simulink model "DrivetrainConVeh"  (R2024a)
settings: Solver=ode23tb  StartTime=0.0  StopTime=50  RelTol=1e-3  EnableMultiTasking=on
model workspace (MAT data in the model file):
  N : Simulink.Parameter (value not decoded)
  NF : Simulink.Parameter (value not decoded)
  NR : Simulink.Parameter (value not decoded)
  Ndiff : Simulink.Parameter (value not decoded)
  RWheel : Simulink.Parameter (value not decoded)
  b_axle : Simulink.Parameter (value not decoded)
  b_driveshaft : Simulink.Parameter (value not decoded)
  dt_DCT : Simulink.Parameter (value not decoded)
  k_axle : Simulink.Parameter (value not decoded)
  k_driveshaft : Simulink.Parameter (value not decoded)
  k_hyd : Simulink.Parameter (value not decoded)
  tau_hyd : Simulink.Parameter (value not decoded)
  wc_shaft : Simulink.Parameter (value not decoded)
symbols that are objects in the model workspace (value not decoded): b_axle, b_driveshaft, k_axle, k_driveshaft, k_hyd, N, tau_hyd
libraries: autolibsharedcoupling x12, autolibpowerinfoutils x6, autolibshareddiff x5, autolibutils x3, autolibshared x3, autolibcoupling x2, simulink x2, autolibsharedtransfixedgear x2, autolibtransdct x1, autolibshareddrivetraincommon x1, autolibtranscontrols x1
(part 3 of 4)

== system DrivetrainConVeh/DCT/DCT Block ==
  GearReq : Inport
  Tin : Inport  Port=2
  Driveshaft Compliance : autolibsharedcoupling/Torsional Compliance  port_config=Two-way connection  extInfo=off  k=k_driveshaft  b=b_driveshaft  theta_o=0  domega_o=0  omega_c=wc_shaft  blkID=0  aMode=1
  Dual Clutch Transmission : autolibtransdct/Dual Clutch Transmission  VariantControl=0  cntrlType=Ideal integrated controller  TransEffModelPopup=Gear only  Jin=0.2  bin=.001  omegain_o=0  G=[-1, 0, 1, 2, 3, 4, 5, 6, 7, 8]  Trq_bpts=[25 50 75 100 150 200 250]  omega_bpts=[52.4 78.5 105 131 157 183 209 262 314 419 524]  Temp_bpts=[313 358]  N=N  Jout=[0.28 0.28 0.28 0.24 0.2 0.18 0.11 0.11 0.11 0.11]  bout=[.001 .001 .001 .0025 .002 .001 .001 .001 .001 .001]  eta=[0.930, 0.930, 0.930, 0.940,0.947, 0.948,0.946, 0.943,0.940, 0.935 ]  eta_tbl=reshape([0.57 0.77 0.83 0.86 0.89 0.89 0.89 0.55 0.76 0.83 0.86 0.89 0.89 0.89 0.59 0.78 0.85 0.88 0.9 0.89 0.89 0.61 0.79 0.85 0.88 0.91 0.89 0.89 0.62 0.8 0.86 0.89 0.91 0.89 0.89 0.62 0.8 0.85 0.89 0.91 0.89 0.89 0.63 0.8 0.86 0.89 0.92 0.89 0.89 0.63 0.8 0.86 0.89 0.92 0.89 0.89 0.62 0.81 0.86 0.89 0.92 0.89 0.89 0.6 0.79 0.85 0.88 0.92 0.89 0.89 0.55 0.77 0.84 0.87 0.91 0.89 0.89 0.57 0.77 0.83 0.86 0.89 0.89 0.89 0.55 0.76 0.83 0.86 0.89 0.89 0.89 0.59 0.78 0.85 0.88 0.9 0.89 0.89 0.61 0.79 0.85 0.88 0.91 0.89 0.89 0.62 0.8 0.86 0.89 0.91 0.89 0.89 0.62 0.8 0.85 0.89 0.91 0.89 0.89 0.63 0.8 0.86 0.89 0.92 0.89 0.89 0.63 0.8 0.86 0.89 0.92 0.89 0.89 0.62 0.81 0.86 0.89 0.92 0.89 0.89 0.6 0.79 0.85 0.88 0.92 0.89 0.89 0.55 0.77 0.84 0.87 0.91 0.89 0.89 0.57 0.77 0.83 0.86 0.89 0.89 0.89 0.55 0.76 0.83 0.86 0.89 0.89 0.89 0.59 0.78 0.85 0.88 0.9 0.89 0.89 0.61 0.79 0.85 0.88 0.91 0.89 0.89 0.62 0.8 0.86 0.89 0.91 0.89 0.89 0.62 0.8 0.85 0.89 0.91 0.89 0.89 0.63 0.8 0.86 0.89 0.92 0.89 0.89 0.63 0.8 0.86 0.89 0.92 0.89 0.89 0.62 0.81 0.86 0.89 0.92 0.89 0.89 0.6 0.79 0.85 0.88 0.92 0.89 0.89 0.55 0.77 0.84 0.87 0.91 0.89 0.89 0.76 0.87 0.9 0.91 0.93 0.92 0.92 0.69 0.83 0.88 0.9 0.91 0.92 0.92 0.64 0.81 0.87 0.89 0.91 0.92 0.92 0.63 0.81 0.86 0.89 0.91 0.92 0.92 0.63 0.81 0.86 0.89 0.92 0.92 0.92 0.62 0.8 0.86 0.89 0.92 0.93 0.92 0.62 0.8 0.86 0.89 0.92 0.93 0.92 0.61 0.8 0.86 0.89 0.92 0.93 0.92 0.61 0.8 0.86 0.89 0.92 0.93 0.92 0.57 0.78 0.84 0.88 0.91 0.93 0.92 0.52 0.76 0.83 0.87 0.91 0.93 0.92 0.71 0.84 0.89 0.9 0.92 0.93 0.93 0.62 0.8 0.86 0.89 0.91 0.92 0.93 0.59 0.79 0.85 0.88 0.91 0.92 0.93 0.58 0.79 0.85 0.88 0.91 0.93 0.93 0.57 0.78 0.85 0.88 0.91 0.93 0.94 0.57 0.78 0.85 0.88 0.91 0.93 0.94 0.57 0.78 0.84 0.88 0.91 0.93 0.94 0.55 0.76 0.84 0.87 0.91 0.93 0.94 0.5 0.75 0.83 0.86 0.9 0.92 0.93 0.48 0.74 0.82 0.86 0.9 0.92 0.93 0.41 0.7 0.79 0.83 0.89 0.91 0.92 0.68 0.83 0.88 0.89 0.92 0.93 0.94 0.59 0.78 0.85 0.87 0.9 0.92 0.93 0.54 0.76 0.83 0.87 0.9 0.92 0.93 0.53 0.76 0.83 0.87 0.9 0.92 0.93 0.51 0.75 0.82 0.86 0.9 0.92 0.93 0.5 0.74 0.82 0.86 0.9 0.92 0.93 0.48 0.72 0.81 0.85 0.89 0.91 0.92 0.42 0.7 0.79 0.84 0.88 0.91 0.92 0.31 0.67 0.77 0.82 0.87 0.9 0.91 0.18 0.57 0.7 0.77 0.84 0.87 0.89 0.094 0.47 0.63 0.72 0.81 0.85 0.87 0.68 0.82 0.88 0.89 0.92 0.93 0.93 0.59 0.78 0.84 0.87 0.9 0.92 0.93 0.54 0.76 0.83 0.86 0.9 0.92 0.92 0.53 0.75 0.83 0.86 0.9 0.92 0.93 0.51 0.75 0.82 0.86 0.9 0.92 0.93 0.49 0.74 0.82 0.85 0.89 0.91 0.92 0.47 0.72 0.8 0.85 0.89 0.91 0.92 0.42 0.7 0.79 0.84 0.88 0.9 0.92 0.31 0.67 0.76 0.82 0.87 0.9 0.91 0.18 0.57 0.7 0.77 0.84 0.87 0.89 0.094 0.47 0.63 0.72 0.8 0.85 0.87 0.68 0.82 0.87 0.89 0.91 0.92 0.93 0.59 0.78 0.84 0.87 0.9 0.92 0.93 0.54 0.75 0.83 0.86 0.9 0.91 0.92 0.53 0.75 0.82 0.86 0.9 0.91 0.92 0.51 0.74 0.82 0.86 0.89 0.91 0.92 0.49 0.73 0.81 0.85 0.89 0.91 0.92 0.47 0.72 0.8 0.85 0.89 0.91 0.92 0.42 0.7 0.78 0.83 0.88 0.9 0.91 0.31 0.66 0.76 0.81 0.87 0.89 0.91 0.18 0.57 0.7 0.77 0.83 0.87 0.89 0.093 0.46 0.63 0.72 0.8 0.84 0.87 0.68 0.82 0.87 0.89 0.91 0.92 0.93 0.58 0.78 0.84 0.87 0.9 0.91 0.92 0.54 0.75 0.82 0.86 0.89 0.91 0.92 0.53 0.75 0.82 0.86 0.89 0.91 0.92 0.51 0.74 0.81 0.85 0.89 0.91 0.92 0.49 0.73 0.81 0.85 0.89 0.91 0.92 0.47 0.72 0.8 0.85 0.89 0.91 0.92 0.42 0.69 0.78 0.83 0.88 0.9 0.91 0.31 0.66 0.76 0.81 0.86 0.89 0.9 0.18 0.57 0.69 0.76 0.83 0.87 0.89 0.093 0.46 0.63 0.71 0.8 0.84 0.87 0.67 0.82 0.86 0.88 0.91 0.92 0.92 0.58 0.77 0.83 0.86 0.89 0.91 0.92 0.53 0.75 0.82 0.85 0.89 0.9 0.91 0.52 0.75 0.82 0.85 0.89 0.91 0.92 0.51 0.74 0.81 0.85 0.89 0.91 0.92 0.49 0.73 0.81 0.84 0.88 0.9 0.91 0.47 0.71 0.79 0.84 0.88 0.9 0.91 0.41 0.69 0.78 0.83 0.87 0.89 0.91 0.31 0.66 0.75 0.81 0.86 0.89 0.9 0.18 0.56 0.69 0.76 0.83 0.86 0.88 0.092 0.46 0.63 0.71 0.79 0.84 0.86 0.81 0.88 0.9 0.91 0.92 0.92 0.92 0.75 0.86 0.89 0.91 0.92 0.92 0.92 0.74 0.86 0.89 0.91 0.92 0.92 0.92 0.74 0.86 0.9 0.91 0.93 0.92 0.92 0.74 0.86 0.9 0.91 0.93 0.92 0.92 0.73 0.86 0.89 0.91 0.93 0.92 0.92 ...(+3589 chars))  omegaout_o=0  G_o=0  tauc=.01  ts=.05  tc=.5  R=.25  K_c=2.5e3  mus=0.3  muk=0.25  ClutchLocked=off  SynchLocked=off  maxAbsSpd=5e3
  Two-Way Connection2 : TwoWayConnection
  T : PMIOPort  Side=Right
  Info : Outport  VectorParamsAs1DForOutWhenUnconnected=off
  EngSpd : Outport  Port=2  VectorParamsAs1DForOutWhenUnconnected=off
  wires:
  Dual Clutch Transmission/1 -> Info/1
  Dual Clutch Transmission/2 -> EngSpd/1
  GearReq/1 -> Dual Clutch Transmission/1
  Dual Clutch Transmission/3 -> Two-Way Connection2/1
  Tin/1 -> Dual Clutch Transmission/2
  Two-Way Connection2/1 -> Dual Clutch Transmission/3
  connections:
  T/RConn1 -- Driveshaft Compliance/RConn1
  Driveshaft Compliance/LConn1 -- Two-Way Connection2/RConn1

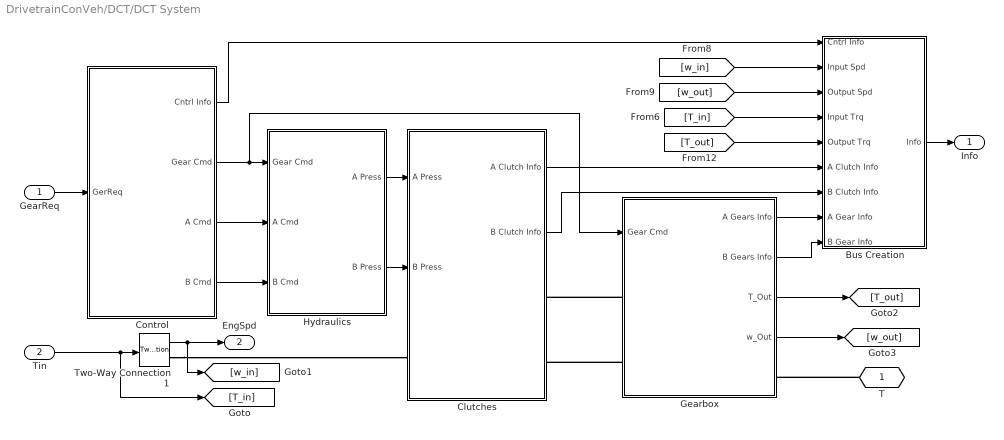
== system DrivetrainConVeh/DCT/DCT System ==
  GearReq : Inport
  Tin : Inport  Port=2  Unit=N*m
  Bus Creation : Subsystem
  Clutches : Subsystem
  Control : Subsystem
  Gearbox : Subsystem
  Hydraulics : Subsystem
  Two-Way Connection1 : TwoWayConnection
  T : PMIOPort  Side=Right
  Info : Outport  VectorParamsAs1DForOutWhenUnconnected=off
  EngSpd : Outport  Port=2  Unit=rad/s  VectorParamsAs1DForOutWhenUnconnected=off
  wires:
  Tin/1 -> [T_in], Two-Way Connection1/1
  Two-Way Connection1/1 -> [w_in], EngSpd/1
  Gearbox/1(A Gears Info) -> Bus Creation/8(A Gear Info)
  Gearbox/2(B Gears Info) -> Bus Creation/9(B Gear Info)
  Clutches/1(A Clutch Info) -> Bus Creation/6(A Clutch Info)
  Clutches/2(B Clutch Info) -> Bus Creation/7(B Clutch Info)
  Hydraulics/1(A Press) -> Clutches/1(A Press)
  Hydraulics/2(B Press) -> Clutches/2(B Press)
  Control/2(Gear Cmd) -> Hydraulics/1(Gear Cmd), Gearbox/1(Gear Cmd)
  GearReq/1 -> Control/1(GerReq)
  Control/3(A Cmd) -> Hydraulics/2(A Cmd)
  Control/4(B Cmd) -> Hydraulics/3(B Cmd)
  [T_out] -> Bus Creation/5(Output Trq)
  [T_in] -> Bus Creation/4(Input Trq)
  Control/1(Cntrl Info) -> Bus Creation/1(Cntrl Info)
  [w_out] -> Bus Creation/3(Output Spd)
  [w_in] -> Bus Creation/2(Input Spd)
  Bus Creation/1(Info) -> Info/1
  Gearbox/3(T_Out) -> [T_out]
  Gearbox/4(w_Out) -> [w_out]
  connections:
  T/RConn1 -- Gearbox/RConn1
  Gearbox/LConn1 -- Clutches/RConn1
  Two-Way Connection1/RConn1 -- Clutches/LConn1
  Gearbox/LConn2 -- Clutches/RConn2

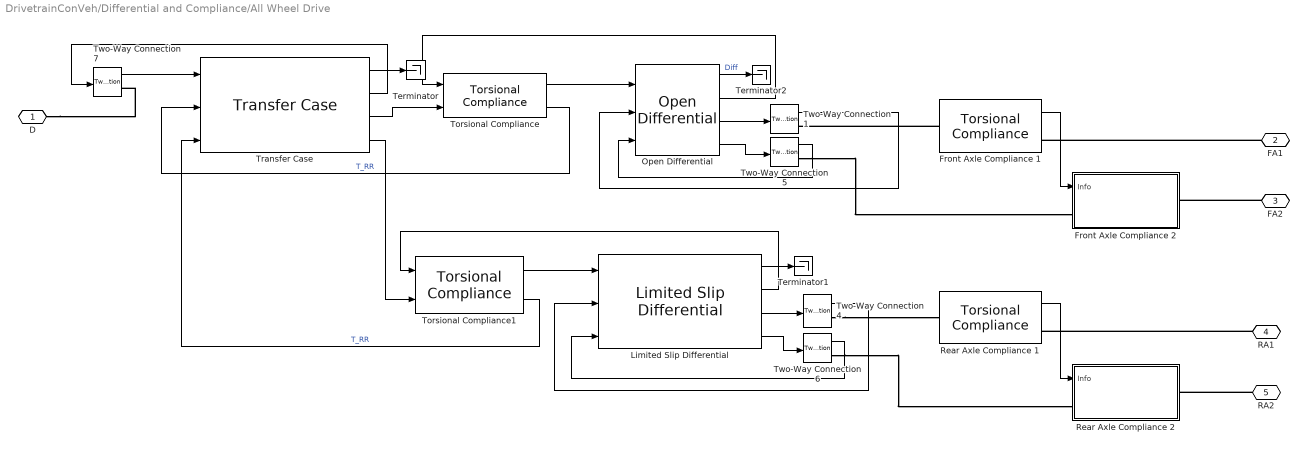
== system DrivetrainConVeh/Differential and Compliance/All Wheel Drive ==
  Front Axle Compliance 1 : autolibsharedcoupling/Torsional Compliance  port_config=Two-way connection  extInfo=on  k=k_axle  b=b_axle  theta_o=0  domega_o=0  omega_c=wc_shaft  blkID=0  aMode=1
  Front Axle Compliance 2 : Subsystem
  Limited Slip Differential : autolibshareddiff/Limited Slip Differential  DiffEffModelPopup=Constant  InterpMethod=Linear point-slope  extTamb=off  shaftSwitchMask=To the left of center-line  Ndiff=Ndiff  Jd=.025  bd=1e-3  Jw1=.01  bw1=1e-3  Jw2=.01  bw2=1e-3  omegaw1o=0  omegaw2o=0  eta=1  eta_tbl=reshape([0.64 0.76 0.8 0.81 0.83 0.84 0.84 0.56 0.73 0.78 0.8 0.83 0.84 0.84 0.54 0.71 0.77 0.8 0.82 0.84 0.84 0.53 0.71 0.77 0.8 0.83 0.84 0.84 0.51 0.71 0.77 0.8 0.83 0.84 0.85 0.52 0.7 0.77 0.8 0.83 0.84 0.85 0.51 0.71 0.76 0.79 0.83 0.84 0.85 0.5 0.69 0.76 0.79 0.82 0.84 0.85 0.45 0.68 0.75 0.78 0.82 0.84 0.85 0.43 0.67 0.74 0.78 0.81 0.83 0.84 0.38 0.63 0.71 0.75 0.8 0.82 0.83 0.81 0.86 0.88 0.89 0.89 0.89 0.9 0.77 0.85 0.87 0.88 0.89 0.9 0.9 0.72 0.82 0.86 0.87 0.88 0.89 0.9 0.68 0.8 0.84 0.86 0.88 0.89 0.89 0.67 0.8 0.84 0.86 0.88 0.89 0.9 0.67 0.8 0.84 0.86 0.88 0.89 0.9 0.65 0.8 0.84 0.86 0.88 0.89 0.9 0.64 0.79 0.83 0.86 0.88 0.89 0.9 0.63 0.78 0.83 0.86 0.88 0.89 0.9 0.59 0.76 0.82 0.85 0.87 0.89 0.9 0.53 0.73 0.8 0.83 0.86 0.88 0.89], 7, 11, 2)  Trq_bpts=[25, 50, 75, 100, 150, 200, 250]  omega_bpts=[52.4 78.5 105 131 157 183 209 262 314 419 524]  Temp_bpts=[290 358]  Tamb=297.15  couplingType=Pre-loaded ideal clutch  Ndisks=4  Reff=.20  Fc=500  muc=[.16 0.13 0.115 0.11 0.105 0.1025 0.10125]  dw=[0 10 20 40 60 80 100]  Tdw=[-100, -90, -50, -5, 0, 5, 50, 90, 100]  dwT=[-200, -175, -100, - 50, 0, 50, 100, 175, 200]  TTin=[-200 -175 -100 - 50 0 50 100 175 200]  Tin=[-200 -175 -100 - 50 0 50 100 175 200]  tauC=.01  IdealInterpMethod=Linear point-slope  IdealExtrapMethod=Linear  TdwInterpMethod=Linear point-slope  TdwExtrapMethod=Linear  TTinInterpMethod=Linear point-slope  TTinExtrapMethod=Linear  maxAbsSpd=5e3  aMode=1
      settings: LibrarySourceBlock=autolibdiff/Limited Slip Differential
  Open Differential : autolibshareddiff/Open Differential  DiffEffModelPopup=Constant  InterpMethod=Linear point-slope  extTamb=off  shaftSwitchMask=To the left of center-line  Ndiff=Ndiff  Jd=.025  bd=1e-3  Jw1=.01  bw1=1e-3  Jw2=.01  bw2=1e-3  omegaw1o=0  omegaw2o=0  eta=1  eta_tbl=reshape([0.64 0.76 0.8 0.81 0.83 0.84 0.84 0.56 0.73 0.78 0.8 0.83 0.84 0.84 0.54 0.71 0.77 0.8 0.82 0.84 0.84 0.53 0.71 0.77 0.8 0.83 0.84 0.84 0.51 0.71 0.77 0.8 0.83 0.84 0.85 0.52 0.7 0.77 0.8 0.83 0.84 0.85 0.51 0.71 0.76 0.79 0.83 0.84 0.85 0.5 0.69 0.76 0.79 0.82 0.84 0.85 0.45 0.68 0.75 0.78 0.82 0.84 0.85 0.43 0.67 0.74 0.78 0.81 0.83 0.84 0.38 0.63 0.71 0.75 0.8 0.82 0.83 0.81 0.86 0.88 0.89 0.89 0.89 0.9 0.77 0.85 0.87 0.88 0.89 0.9 0.9 0.72 0.82 0.86 0.87 0.88 0.89 0.9 0.68 0.8 0.84 0.86 0.88 0.89 0.89 0.67 0.8 0.84 0.86 0.88 0.89 0.9 0.67 0.8 0.84 0.86 0.88 0.89 0.9 0.65 0.8 0.84 0.86 0.88 0.89 0.9 0.64 0.79 0.83 0.86 0.88 0.89 0.9 0.63 0.78 0.83 0.86 0.88 0.89 0.9 0.59 0.76 0.82 0.85 0.87 0.89 0.9 0.53 0.73 0.8 0.83 0.86 0.88 0.89], 7, 11, 2)  Trq_bpts=[25, 50, 75, 100, 150, 200, 250]  omega_bpts=[52.4 78.5 105 131 157 183 209 262 314 419 524]  Temp_bpts=[290 358]  Tamb=297.15  maxAbsSpd=5e3  aMode=1
      settings: LibrarySourceBlock=autolibdiff/Open Differential
  Rear Axle Compliance 1 : autolibsharedcoupling/Torsional Compliance  port_config=Two-way connection  extInfo=on  k=k_axle  b=b_axle  theta_o=0  domega_o=0  omega_c=wc_shaft  blkID=0  aMode=1
  Rear Axle Compliance 2 : Subsystem
  Terminator : Terminator
  Terminator1 : Terminator
  Terminator2 : Terminator
  Torsional Compliance : autolibsharedcoupling/Torsional Compliance  port_config=Simulink  extInfo=off  k=1e4  b=1e2  theta_o=0  domega_o=0  omega_c=3000  blkID=0  aMode=1
  Torsional Compliance1 : autolibsharedcoupling/Torsional Compliance  port_config=Simulink  extInfo=off  k=1e4  b=1e2  theta_o=0  domega_o=0  omega_c=3000  blkID=0  aMode=1
  Transfer Case : autolibshareddiff/Transfer Case  DiffEffModelPopup=Constant  InterpMethod=Linear point-slope  extTamb=off  TrqSplitRatioMode=off  SpdLockMode=off  shaftSwitchMask=To the left of center-line  Ndiff=1  Jd=.1  bd=1e-3  Jw1=.1  bw1=1e-3  Jw2=.1  bw2=1e-3  omegaw1o=0  omegaw2o=0  eta=1  eta_tbl=reshape([0.64 0.76 0.8 0.81 0.83 0.84 0.84 0.56 0.73 0.78 0.8 0.83 0.84 0.84 0.54 0.71 0.77 0.8 0.82 0.84 0.84 0.53 0.71 0.77 0.8 0.83 0.84 0.84 0.51 0.71 0.77 0.8 0.83 0.84 0.85 0.52 0.7 0.77 0.8 0.83 0.84 0.85 0.51 0.71 0.76 0.79 0.83 0.84 0.85 0.5 0.69 0.76 0.79 0.82 0.84 0.85 0.45 0.68 0.75 0.78 0.82 0.84 0.85 0.43 0.67 0.74 0.78 0.81 0.83 0.84 0.38 0.63 0.71 0.75 0.8 0.82 0.83 0.81 0.86 0.88 0.89 0.89 0.89 0.9 0.77 0.85 0.87 0.88 0.89 0.9 0.9 0.72 0.82 0.86 0.87 0.88 0.89 0.9 0.68 0.8 0.84 0.86 0.88 0.89 0.89 0.67 0.8 0.84 0.86 0.88 0.89 0.9 0.67 0.8 0.84 0.86 0.88 0.89 0.9 0.65 0.8 0.84 0.86 0.88 0.89 0.9 0.64 0.79 0.83 0.86 0.88 0.89 0.9 0.63 0.78 0.83 0.86 0.88 0.89 0.9 0.59 0.76 0.82 0.85 0.87 0.89 0.9 0.53 0.73 0.8 0.83 0.86 0.88 0.89], 7, 11, 2)  Trq_bpts=[25, 50, 75, 100, 150, 200, 250]  omega_bpts=[52.4 78.5 105 131 157 183 209 262 314 419 524]  Temp_bpts=[290 358]  Tamb=297.15  maxAbsSpd=5e3  aMode=1  TrqSplitRatio=0.5  SpdLock=0
      settings: LibrarySourceBlock=autolibdiff/Transfer Case
  Two-Way Connection{1,4..7} (5 alike) : TwoWayConnection
  D : PMIOPort  Side=Left
  FA1 : PMIOPort  Port=2  Side=Right
  FA2 : PMIOPort  Port=3  Side=Right
  RA1 : PMIOPort  Port=4  Side=Right
  RA2 : PMIOPort  Port=5  Side=Right
  wires:
  Open Differential/1 -> Terminator2/1  "Diff"
  Two-Way Connection1/1 -> Open Differential/2
  Open Differential/3 -> Two-Way Connection1/1
  Open Differential/2 -> Torsional Compliance/1
  Limited Slip Differential/1 -> Terminator1/1
  Limited Slip Differential/3 -> Two-Way Connection4/1
  Two-Way Connection4/1 -> Limited Slip Differential/2
  Front Axle Compliance 1/1 -> Front Axle Compliance 2/1(Info)
  Open Differential/4 -> Two-Way Connection5/1
  Two-Way Connection5/1 -> Open Differential/3
  Rear Axle Compliance 1/1 -> Rear Axle Compliance 2/1(Info)
  Limited Slip Differential/4 -> Two-Way Connection6/1
  Two-Way Connection6/1 -> Limited Slip Differential/3
  Two-Way Connection7/1 -> Transfer Case/1
  Transfer Case/1 -> Terminator/1
  Transfer Case/2 -> Two-Way Connection7/1
  Transfer Case/3 -> Torsional Compliance/2
  Transfer Case/4 -> Torsional Compliance1/2
  Limited Slip Differential/2 -> Torsional Compliance1/1
  Torsional Compliance1/1 -> Limited Slip Differential/1
  Torsional Compliance/1 -> Open Differential/1
  Torsional Compliance/2 -> Transfer Case/2  "T_RR"
  Torsional Compliance1/2 -> Transfer Case/3  "T_RR"
  connections:
  D/RConn1 -- Two-Way Connection7/RConn1
  Two-Way Connection5/RConn1 -- Front Axle Compliance 2/LConn1
  FA2/RConn1 -- Front Axle Compliance 2/RConn1
  FA1/RConn1 -- Front Axle Compliance 1/RConn1
  Front Axle Compliance 1/LConn1 -- Two-Way Connection1/RConn1
  RA2/RConn1 -- Rear Axle Compliance 2/RConn1
  Two-Way Connection4/RConn1 -- Rear Axle Compliance 1/LConn1
  RA1/RConn1 -- Rear Axle Compliance 1/RConn1
  Two-Way Connection6/RConn1 -- Rear Axle Compliance 2/LConn1

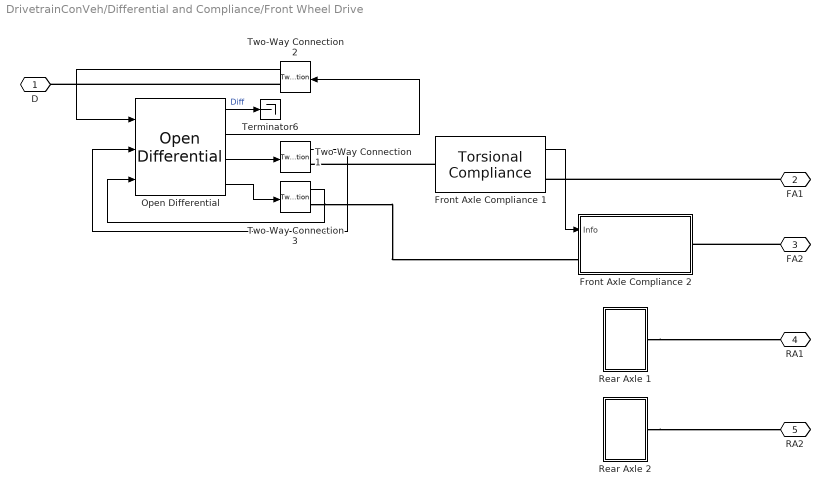
== system DrivetrainConVeh/Differential and Compliance/Front Wheel Drive ==
  Front Axle Compliance 1 : autolibsharedcoupling/Torsional Compliance  port_config=Two-way connection  extInfo=on  k=k_axle  b=b_axle  theta_o=0  domega_o=0  omega_c=wc_shaft  blkID=0  aMode=1
  Front Axle Compliance 2 : Subsystem
  Open Differential : autolibshareddiff/Open Differential  DiffEffModelPopup=Constant  InterpMethod=Linear point-slope  extTamb=off  shaftSwitchMask=To the left of center-line  Ndiff=Ndiff  Jd=.025  bd=1e-3  Jw1=.01  bw1=1e-3  Jw2=.01  bw2=1e-3  omegaw1o=0  omegaw2o=0  eta=1  eta_tbl=reshape([0.64 0.76 0.8 0.81 0.83 0.84 0.84 0.56 0.73 0.78 0.8 0.83 0.84 0.84 0.54 0.71 0.77 0.8 0.82 0.84 0.84 0.53 0.71 0.77 0.8 0.83 0.84 0.84 0.51 0.71 0.77 0.8 0.83 0.84 0.85 0.52 0.7 0.77 0.8 0.83 0.84 0.85 0.51 0.71 0.76 0.79 0.83 0.84 0.85 0.5 0.69 0.76 0.79 0.82 0.84 0.85 0.45 0.68 0.75 0.78 0.82 0.84 0.85 0.43 0.67 0.74 0.78 0.81 0.83 0.84 0.38 0.63 0.71 0.75 0.8 0.82 0.83 0.81 0.86 0.88 0.89 0.89 0.89 0.9 0.77 0.85 0.87 0.88 0.89 0.9 0.9 0.72 0.82 0.86 0.87 0.88 0.89 0.9 0.68 0.8 0.84 0.86 0.88 0.89 0.89 0.67 0.8 0.84 0.86 0.88 0.89 0.9 0.67 0.8 0.84 0.86 0.88 0.89 0.9 0.65 0.8 0.84 0.86 0.88 0.89 0.9 0.64 0.79 0.83 0.86 0.88 0.89 0.9 0.63 0.78 0.83 0.86 0.88 0.89 0.9 0.59 0.76 0.82 0.85 0.87 0.89 0.9 0.53 0.73 0.8 0.83 0.86 0.88 0.89], 7, 11, 2)  Trq_bpts=[25, 50, 75, 100, 150, 200, 250]  omega_bpts=[52.4 78.5 105 131 157 183 209 262 314 419 524]  Temp_bpts=[290 358]  Tamb=297.15  maxAbsSpd=5e3  aMode=1
      settings: LibrarySourceBlock=autolibdiff/Open Differential
  Rear Axle 1 : Subsystem
  Rear Axle 2 : Subsystem
  Terminator6 : Terminator
  Two-Way Connection1 : TwoWayConnection
  Two-Way Connection2 : TwoWayConnection
  Two-Way Connection3 : TwoWayConnection
  D : PMIOPort  Side=Left
  FA1 : PMIOPort  Port=2  Side=Right
  FA2 : PMIOPort  Port=3  Side=Right
  RA1 : PMIOPort  Port=4  Side=Right
  RA2 : PMIOPort  Port=5  Side=Right
  wires:
  Open Differential/1 -> Terminator6/1  "Diff"
  Two-Way Connection2/1 -> Open Differential/1
  Two-Way Connection1/1 -> Open Differential/2
  Open Differential/3 -> Two-Way Connection1/1
  Open Differential/2 -> Two-Way Connection2/1
  Front Axle Compliance 1/1 -> Front Axle Compliance 2/1(Info)
  Open Differential/4 -> Two-Way Connection3/1
  Two-Way Connection3/1 -> Open Differential/3
  connections:
  FA1/RConn1 -- Front Axle Compliance 1/RConn1
  Front Axle Compliance 1/LConn1 -- Two-Way Connection1/RConn1
  Two-Way Connection2/RConn1 -- D/RConn1
  Two-Way Connection3/RConn1 -- Front Axle Compliance 2/LConn1
  FA2/RConn1 -- Front Axle Compliance 2/RConn1
  Rear Axle 1/RConn1 -- RA1/RConn1
  Rear Axle 2/RConn1 -- RA2/RConn1

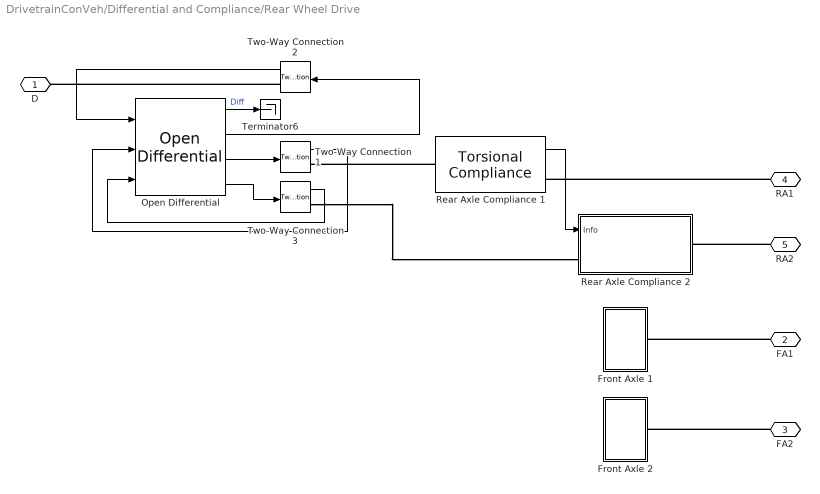
== system DrivetrainConVeh/Differential and Compliance/Rear Wheel Drive ==
  Front Axle 1 : Subsystem
  Front Axle 2 : Subsystem
  Open Differential : autolibshareddiff/Open Differential  DiffEffModelPopup=Constant  InterpMethod=Linear point-slope  extTamb=off  shaftSwitchMask=To the left of center-line  Ndiff=Ndiff  Jd=.025  bd=1e-3  Jw1=.01  bw1=1e-3  Jw2=.01  bw2=1e-3  omegaw1o=0  omegaw2o=0  eta=1  eta_tbl=reshape([0.64 0.76 0.8 0.81 0.83 0.84 0.84 0.56 0.73 0.78 0.8 0.83 0.84 0.84 0.54 0.71 0.77 0.8 0.82 0.84 0.84 0.53 0.71 0.77 0.8 0.83 0.84 0.84 0.51 0.71 0.77 0.8 0.83 0.84 0.85 0.52 0.7 0.77 0.8 0.83 0.84 0.85 0.51 0.71 0.76 0.79 0.83 0.84 0.85 0.5 0.69 0.76 0.79 0.82 0.84 0.85 0.45 0.68 0.75 0.78 0.82 0.84 0.85 0.43 0.67 0.74 0.78 0.81 0.83 0.84 0.38 0.63 0.71 0.75 0.8 0.82 0.83 0.81 0.86 0.88 0.89 0.89 0.89 0.9 0.77 0.85 0.87 0.88 0.89 0.9 0.9 0.72 0.82 0.86 0.87 0.88 0.89 0.9 0.68 0.8 0.84 0.86 0.88 0.89 0.89 0.67 0.8 0.84 0.86 0.88 0.89 0.9 0.67 0.8 0.84 0.86 0.88 0.89 0.9 0.65 0.8 0.84 0.86 0.88 0.89 0.9 0.64 0.79 0.83 0.86 0.88 0.89 0.9 0.63 0.78 0.83 0.86 0.88 0.89 0.9 0.59 0.76 0.82 0.85 0.87 0.89 0.9 0.53 0.73 0.8 0.83 0.86 0.88 0.89], 7, 11, 2)  Trq_bpts=[25, 50, 75, 100, 150, 200, 250]  omega_bpts=[52.4 78.5 105 131 157 183 209 262 314 419 524]  Temp_bpts=[290 358]  Tamb=297.15  maxAbsSpd=5e3  aMode=1
      settings: LibrarySourceBlock=autolibdiff/Open Differential
  Rear Axle Compliance 1 : autolibsharedcoupling/Torsional Compliance  port_config=Two-way connection  extInfo=on  k=k_axle  b=b_axle  theta_o=0  domega_o=0  omega_c=wc_shaft  blkID=0  aMode=1
  Rear Axle Compliance 2 : Subsystem
  Terminator6 : Terminator
  Two-Way Connection1 : TwoWayConnection
  Two-Way Connection2 : TwoWayConnection
  Two-Way Connection3 : TwoWayConnection
  D : PMIOPort  Side=Left
  FA1 : PMIOPort  Port=2  Side=Right
  FA2 : PMIOPort  Port=3  Side=Right
  RA1 : PMIOPort  Port=4  Side=Right
  RA2 : PMIOPort  Port=5  Side=Right
  wires:
  Two-Way Connection3/1 -> Open Differential/3
  Open Differential/4 -> Two-Way Connection3/1
  Open Differential/2 -> Two-Way Connection2/1
  Two-Way Connection1/1 -> Open Differential/2
  Two-Way Connection2/1 -> Open Differential/1
  Open Differential/1 -> Terminator6/1  "Diff"
  Open Differential/3 -> Two-Way Connection1/1
  Rear Axle Compliance 1/1 -> Rear Axle Compliance 2/1(Info)
  connections:
  Rear Axle Compliance 1/LConn1 -- Two-Way Connection1/RConn1
  Two-Way Connection3/RConn1 -- Rear Axle Compliance 2/LConn1
  Two-Way Connection2/RConn1 -- D/RConn1
  RA1/RConn1 -- Rear Axle Compliance 1/RConn1
  RA2/RConn1 -- Rear Axle Compliance 2/RConn1
  FA1/RConn1 -- Front Axle 1/RConn1
  FA2/RConn1 -- Front Axle 2/RConn1

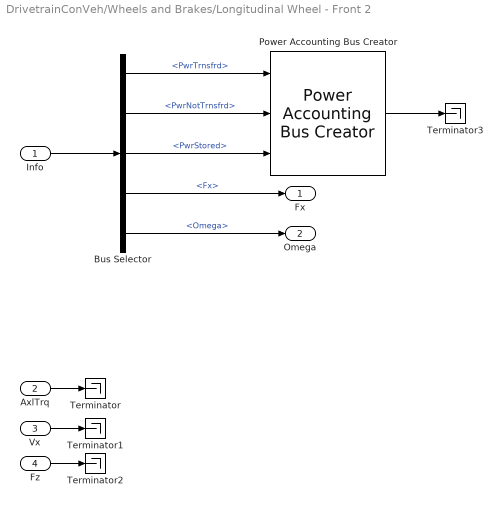
== system DrivetrainConVeh/Wheels and Brakes/Longitudinal Wheel - Front 2 ==
  Info : Inport
  AxlTrq : Inport  Port=2
  Vx : Inport  Port=3
  Fz : Inport  Port=4
  Bus Selector : BusSelector  OutputSignals=PwrInfo.PwrTrnsfrd,PwrInfo.PwrNotTrnsfrd,PwrInfo.PwrStored,Fx,Omega
  Power Accounting Bus Creator : autolibpowerinfoutils/Power Accounting Bus Creator  AssctBlkSelPopup=Parent  RefBlkName='libraryname/blkname'  PwrTrnsfrdCheckBox=on  PwrNotTrnsfrdCheckBox=on  PwrStoredCheckBox=on  aMode=aMode
  Terminator{,1..3} (4 alike) : Terminator
  Fx : Outport  VectorParamsAs1DForOutWhenUnconnected=off
  Omega : Outport  Port=2  VectorParamsAs1DForOutWhenUnconnected=off
  wires:
  AxlTrq/1 -> Terminator/1
  Vx/1 -> Terminator1/1
  Fz/1 -> Terminator2/1
  Info/1 -> Bus Selector/1
  Bus Selector/1 -> Power Accounting Bus Creator/1  "<PwrTrnsfrd>"
  Bus Selector/2 -> Power Accounting Bus Creator/2  "<PwrNotTrnsfrd>"
  Bus Selector/3 -> Power Accounting Bus Creator/3  "<PwrStored>"
  Bus Selector/4 -> Fx/1  "<Fx>"
  Bus Selector/5 -> Omega/1  "<Omega>"
  Power Accounting Bus Creator/1 -> Terminator3/1

== system DrivetrainConVeh/Wheels and Brakes/Longitudinal Wheel - Rear 2 ==
  Info : Inport
  AxlTrq : Inport  Port=2
  Vx : Inport  Port=3
  Fz : Inport  Port=4
  Bus Selector : BusSelector  OutputSignals=PwrInfo.PwrTrnsfrd,PwrInfo.PwrNotTrnsfrd,PwrInfo.PwrStored,Fx,Omega
  Power Accounting Bus Creator : autolibpowerinfoutils/Power Accounting Bus Creator  AssctBlkSelPopup=Parent  RefBlkName='libraryname/blkname'  PwrTrnsfrdCheckBox=on  PwrNotTrnsfrdCheckBox=on  PwrStoredCheckBox=on  aMode=aMode
  Terminator{,1..3} (4 alike) : Terminator
  Fx : Outport  VectorParamsAs1DForOutWhenUnconnected=off
  Omega : Outport  Port=2  VectorParamsAs1DForOutWhenUnconnected=off
  wires:
  AxlTrq/1 -> Terminator/1
  Vx/1 -> Terminator1/1
  Fz/1 -> Terminator2/1
  Info/1 -> Bus Selector/1
  Bus Selector/1 -> Power Accounting Bus Creator/1  "<PwrTrnsfrd>"
  Bus Selector/2 -> Power Accounting Bus Creator/2  "<PwrNotTrnsfrd>"
  Bus Selector/3 -> Power Accounting Bus Creator/3  "<PwrStored>"
  Bus Selector/4 -> Fx/1  "<Fx>"
  Bus Selector/5 -> Omega/1  "<Omega>"
  Power Accounting Bus Creator/1 -> Terminator3/1

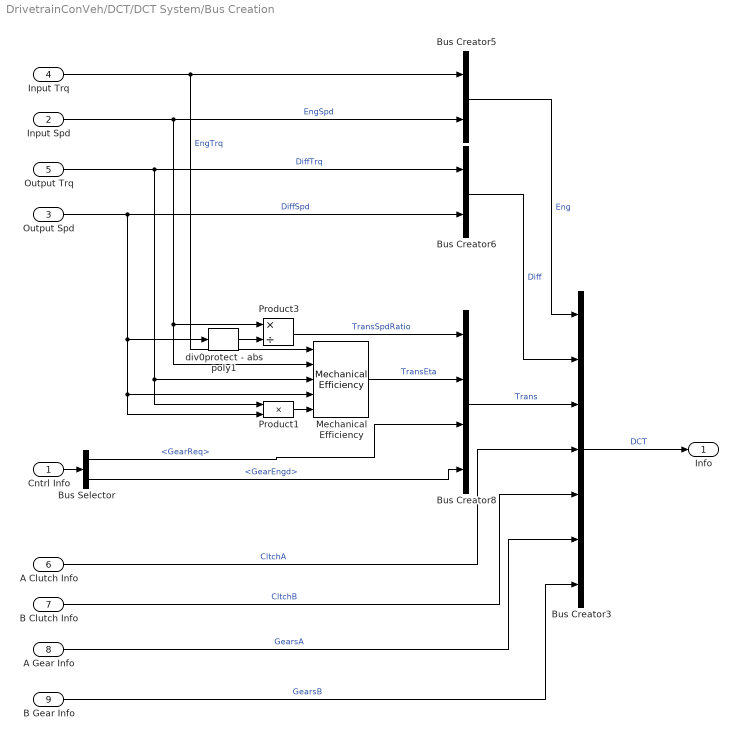
== system DrivetrainConVeh/DCT/DCT System/Bus Creation ==
  Cntrl Info : Inport
  Input Spd : Inport  Port=2  Unit=rad/s
  Output Spd : Inport  Port=3  Unit=rad/s
  Input Trq : Inport  Port=4  Unit=N*m
  Output Trq : Inport  Port=5  Unit=N*m
  A Clutch Info : Inport  Port=6
  B Clutch Info : Inport  Port=7
  A Gear Info : Inport  Port=8
  B Gear Info : Inport  Port=9
  Bus Creator3 : BusCreator  Inputs=7
  Bus Creator5 : BusCreator  Inputs=2
  Bus Creator6 : BusCreator  Inputs=2
  Bus Creator8 : BusCreator  Inputs=4
  Bus Selector : BusSelector  OutputSignals=GearReq,GearEngd
  Mechanical Efficiency : autolibshareddrivetraincommon/Mechanical Efficiency
  Product1 : Product  Inputs=**
  Product3 : Product  Inputs=*/
  div0protect - abs poly1 : autolibutils/div0protect - abs poly  thresh=1e-6  aMode=aMode
  Info : Outport  VectorParamsAs1DForOutWhenUnconnected=off
  wires:
  A Clutch Info/1 -> Bus Creator3/4  "CltchA"
  B Clutch Info/1 -> Bus Creator3/5  "CltchB"
  A Gear Info/1 -> Bus Creator3/6  "GearsA"
  B Gear Info/1 -> Bus Creator3/7  "GearsB"
  Bus Creator3/1 -> Info/1  "DCT"
  Bus Selector/1 -> Bus Creator8/3  "<GearReq>"
  Input Spd/1 -> Bus Creator5/2, Mechanical Efficiency/2, Product3/1  "EngSpd"
  Input Trq/1 -> Bus Creator5/1, Mechanical Efficiency/1  "EngTrq"
  Mechanical Efficiency/1 -> Bus Creator8/2  "TransEta"
  Output Spd/1 -> Bus Creator6/2, Product1/2, Mechanical Efficiency/4, div0protect - abs poly1/1  "DiffSpd"
  Output Trq/1 -> Bus Creator6/1, Product1/1, Mechanical Efficiency/3  "DiffTrq"
  Bus Selector/2 -> Bus Creator8/4  "<GearEngd>"
  Bus Creator8/1 -> Bus Creator3/3  "Trans"
  Product3/1 -> Bus Creator8/1  "TransSpdRatio"
  Product1/1 -> Mechanical Efficiency/5
  Bus Creator6/1 -> Bus Creator3/2  "Diff"
  Bus Creator5/1 -> Bus Creator3/1  "Eng"
  Cntrl Info/1 -> Bus Selector/1
  div0protect - abs poly1/1 -> Product3/2

== system DrivetrainConVeh/DCT/DCT System/Clutches ==
  A Press : Inport
  B Press : Inport  Port=2
  Disc Clutch A : autolibcoupling/Disc Clutch  port_config=Two-way connection  Reff=.25  Ndisk=1  Aeff=.001  Peng=0  Jin=.05  Jout=.001  muk=.25  mus=.3  bin=.001  bout=.001  win_o=0  wout_o=0  tauC=.01  InitiallyLocked=off  maxAbsSpd=3000  blkID=1
  Disc Clutch B : autolibcoupling/Disc Clutch  port_config=Two-way connection  Reff=.25  Ndisk=1  Aeff=.001  Peng=0  Jin=.05  Jout=.001  muk=.25  mus=.3  bin=.001  bout=.001  win_o=0  wout_o=0  tauC=.01  InitiallyLocked=off  maxAbsSpd=3000  blkID=1
  Rotational Inertia : autolibsharedcoupling/Rotational Inertia  port_config=Two-way connection  extInfo=off  externJ=off  J=.1  b=.001  omega_o=0  blkID=0  aMode=1
      settings: LibrarySourceBlock=autolibcoupling/Rotational Inertia
  Split Torsional Compliance : autolibsharedcoupling/Split Torsional Compliance  port_config=Two-way connection  cplrMode=Shaft split  extInfo=off  k1=5e3  b1=50  omega1_c=200  theta1_o=0  domega1_o=0  k2=5e3  b2=50  omega2_c=200  theta2_o=0  domega2_o=0  blkID=0  aMode=1
      settings: LibrarySourceBlock=autolibcoupling/Split Torsional Compliance
  A : PMIOPort  Side=Right
  E : PMIOPort  Port=2  Side=Left
  B : PMIOPort  Port=3  Side=Right
  A Clutch Info : Outport  VectorParamsAs1DForOutWhenUnconnected=off
  B Clutch Info : Outport  Port=2  VectorParamsAs1DForOutWhenUnconnected=off
  wires:
  Disc Clutch B/1 -> B Clutch Info/1
  B Press/1 -> Disc Clutch B/1
  A Press/1 -> Disc Clutch A/1
  Disc Clutch A/1 -> A Clutch Info/1
  connections:
  Split Torsional Compliance/RConn2 -- Disc Clutch B/LConn1
  E/RConn1 -- Rotational Inertia/LConn1
  Split Torsional Compliance/LConn1 -- Rotational Inertia/RConn1
  Split Torsional Compliance/RConn1 -- Disc Clutch A/LConn1
  A/RConn1 -- Disc Clutch A/RConn1
  Disc Clutch B/RConn1 -- B/RConn1

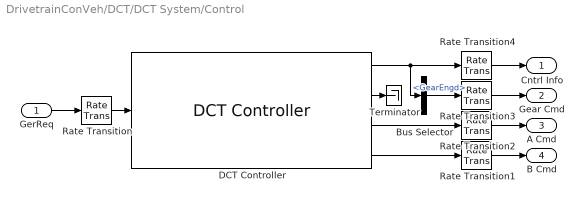
== system DrivetrainConVeh/DCT/DCT System/Control ==
  GerReq : Inport
  Bus Selector : BusSelector  OutputSignals=GearEngd
  DCT Controller : autolibtranscontrols/DCT Controller  G_o=0  tc=.5  ts=.01  dt=dt_DCT  ClutchLocked=off  SynchLocked=off
  Rate Transition : RateTransition  Deterministic=off
  Rate Transition{1..4} (4 alike) : RateTransition
  Terminator : Terminator
  Cntrl Info : Outport  VectorParamsAs1DForOutWhenUnconnected=off
  Gear Cmd : Outport  Port=2  VectorParamsAs1DForOutWhenUnconnected=off
  A Cmd : Outport  Port=3  VectorParamsAs1DForOutWhenUnconnected=off
  B Cmd : Outport  Port=4  VectorParamsAs1DForOutWhenUnconnected=off
  wires:
  DCT Controller/1 -> Bus Selector/1, Rate Transition4/1
  Rate Transition/1 -> DCT Controller/1
  DCT Controller/3 -> Rate Transition2/1
  GerReq/1 -> Rate Transition/1
  DCT Controller/4 -> Rate Transition1/1
  DCT Controller/2 -> Terminator/1
  Rate Transition3/1 -> Gear Cmd/1
  Rate Transition4/1 -> Cntrl Info/1
  Rate Transition1/1 -> B Cmd/1
  Rate Transition2/1 -> A Cmd/1
  Bus Selector/1 -> Rate Transition3/1  "<GearEngd>"

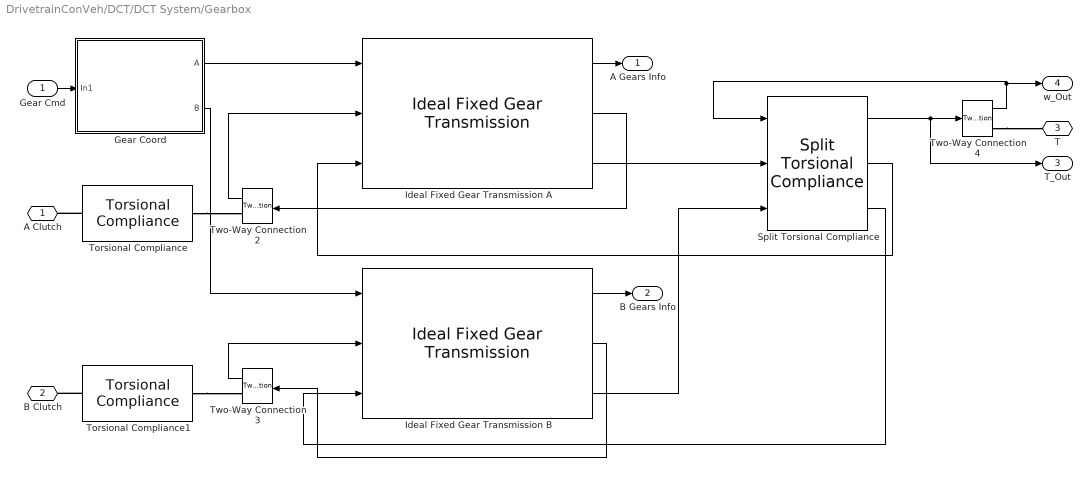
== system DrivetrainConVeh/DCT/DCT System/Gearbox ==
  Gear Cmd : Inport
  Gear Coord : Subsystem
  Ideal Fixed Gear Transmission A : autolibsharedtransfixedgear/Ideal Fixed Gear Transmission  VariantControl=0  TransEffModelPopup=Gear only  gearInterp=Nearest  G=[0,1,3,5,7]  Trq_bpts=[25, 50, 75, 100, 150, 200, 250]  omega_bpts=[52.4 78.5 105 131 157 183 209 262 314 419 524]  Temp_bpts=[313 358]  N=[N(2), N(3:2:end)]  Jout=[0.18 0.28 .2 0.11 0.11]  bout=[.001 .003 .002 .001 .001]  eta=[0.9, 0.9, 0.9, 0.9, 0.9]  eta_tbl=reshape([0.53 0.71 0.77 0.79 0.82 0.82 0.82 0.5 0.7 0.77 0.79 0.82 0.82 0.82 0.54 0.72 0.78 0.81 0.83 0.82 0.82 0.56 0.73 0.79 0.81 0.84 0.82 0.82 0.58 0.74 0.79 0.82 0.84 0.82 0.82 0.57 0.74 0.79 0.82 0.84 0.82 0.82 0.58 0.74 0.79 0.82 0.84 0.82 0.82 0.58 0.74 0.79 0.82 0.84 0.82 0.82 0.57 0.74 0.8 0.82 0.85 0.82 0.82 0.55 0.73 0.78 0.81 0.84 0.82 0.82 0.51 0.71 0.77 0.81 0.84 0.82 0.82 0.53 0.71 0.77 0.79 0.82 0.82 0.82 0.5 0.7 0.77 0.79 0.82 0.82 0.82 0.54 0.72 0.78 0.81 0.83 0.82 0.82 0.56 0.73 0.79 0.81 0.84 0.82 0.82 0.58 0.74 0.79 0.82 0.84 0.82 0.82 0.57 0.74 0.79 0.82 0.84 0.82 0.82 0.58 0.74 0.79 0.82 0.84 0.82 0.82 0.58 0.74 0.79 0.82 0.84 0.82 0.82 0.57 0.74 0.8 0.82 0.85 0.82 0.82 0.55 0.73 0.78 0.81 0.84 0.82 0.82 0.51 0.71 0.77 0.81 0.84 0.82 0.82 0.53 0.71 0.77 0.79 0.82 0.82 0.82 0.5 0.7 0.77 0.79 0.82 0.82 0.82 0.54 0.72 0.78 0.81 0.83 0.82 0.82 0.56 0.73 0.79 0.81 0.84 0.82 0.82 0.58 0.74 0.79 0.82 0.84 0.82 0.82 0.57 0.74 0.79 0.82 0.84 0.82 0.82 0.58 0.74 0.79 0.82 0.84 0.82 0.82 0.58 0.74 0.79 0.82 0.84 0.82 0.82 0.57 0.74 0.8 0.82 0.85 0.82 0.82 0.55 0.73 0.78 0.81 0.84 0.82 0.82 0.51 0.71 0.77 0.81 0.84 0.82 0.82 0.7 0.79 0.82 0.83 0.84 0.84 0.84 0.63 0.76 0.8 0.82 0.83 0.84 0.84 0.58 0.74 0.79 0.81 0.83 0.84 0.84 0.58 0.74 0.79 0.81 0.83 0.84 0.84 0.58 0.74 0.79 0.81 0.84 0.84 0.84 0.57 0.73 0.78 0.81 0.84 0.85 0.84 0.57 0.73 0.79 0.81 0.84 0.85 0.84 0.56 0.73 0.78 0.81 0.83 0.85 0.84 0.55 0.73 0.78 0.81 0.84 0.85 0.84 0.52 0.71 0.77 0.8 0.83 0.85 0.84 0.48 0.69 0.76 0.79 0.83 0.84 0.84 0.64 0.76 0.8 0.81 0.83 0.84 0.84 0.56 0.73 0.78 0.8 0.83 0.84 0.84 0.54 0.71 0.77 0.8 0.82 0.84 0.84 0.53 0.71 0.77 0.8 0.83 0.84 0.84 0.51 0.71 0.77 0.8 0.83 0.84 0.85 0.52 0.7 0.77 0.8 0.83 0.84 0.85 0.51 0.71 0.76 0.79 0.83 0.84 0.85 0.5 0.69 0.76 0.79 0.82 0.84 0.85 0.45 0.68 0.75 0.78 0.82 0.84 0.85 0.43 0.67 0.74 0.78 0.81 0.83 0.84 0.38 0.63 0.71 0.75 0.8 0.82 0.83 0.65 0.79 0.84 0.85 0.88 0.89 0.89 0.56 0.75 0.81 0.83 0.86 0.88 0.89 0.52 0.72 0.79 0.83 0.86 0.88 0.88 0.51 0.72 0.79 0.83 0.86 0.88 0.89 0.49 0.71 0.78 0.82 0.86 0.88 0.89 0.47 0.7 0.78 0.82 0.86 0.87 0.88 0.45 0.69 0.77 0.81 0.85 0.87 0.88 0.4 0.67 0.75 0.8 0.84 0.86 0.88 0.3 0.64 0.73 0.78 0.83 0.86 0.87 0.17 0.55 0.67 0.73 0.8 0.83 0.85 0.089 0.45 0.61 0.69 0.77 0.81 0.83 0.61 0.75 0.82 0.84 0.87 0.87 0.88 0.54 0.73 0.8 0.82 0.86 0.87 0.88 0.51 0.71 0.79 0.82 0.86 0.87 0.88 0.52 0.72 0.79 0.82 0.86 0.87 0.89 0.52 0.72 0.8 0.83 0.86 0.88 0.89 0.53 0.72 0.79 0.82 0.86 0.87 0.89 0.5 0.7 0.78 0.82 0.86 0.88 0.88 0.46 0.69 0.77 0.81 0.85 0.87 0.88 0.4 0.67 0.75 0.8 0.83 0.86 0.88 0.33 0.64 0.73 0.78 0.83 0.85 0.87 0.33 0.64 0.73 0.78 0.83 0.85 0.87 0.78 0.85 0.87 0.88 0.89 0.89 0.89 0.73 0.83 0.86 0.88 0.89 0.89 0.89 0.72 0.83 0.86 0.88 0.89 0.89 0.89 0.72 0.83 0.87 0.89 0.9 0.89 0.89 0.72 0.83 0.87 0.88 0.9 0.89 0.89 0.71 0.83 0.87 0.88 0.9 0.89 0.89 0.71 0.83 0.86 0.88 0.9 0.89 0.89 0.7 0.82 0.86 0.88 0.9 0.89 0.89 0.69 0.82 0.86 0.88 0.9 0.89 0.89 0.67 0.81 0.86 0.88 0.9 0.89 0.89 0.63 0.79 0.85 0.87 0.89 0.89 0.89 0.78 0.85 0.87 0.88 0.89 0.89 0.89 0.73 0.83 0.86 0.88 0.89 0.89 0.89 0.72 0.83 0.86 0.88 0.89 0.89 0.89 0.72 0.83 0.87 0.89 0.9 0.89 0.89 0.72 0.83 0.87 0.88 0.9 0.89 0.89 0.71 0.83 0.87 0.88 0.9 0.89 0.89 0.71 0.83 0.86 0.88 0.9 0.89 0.89 0.7 0.82 0.86 0.88 0.9 0.89 0.89 0.69 0.82 0.86 0.88 0.9 0.89 0.89 0.67 0.81 0.86 0.88 0.9 0.89 0.89 0.63 0.79 0.85 0.87 0.89 0.89 0.89 0.78 0.85 0.87 0.88 0.89 0.89 0.89 0.73 0.83 0.86 0.88 0.89 0.89 0.89 0.72 0.83 0.86 0.88 0.89 0.89 0.89 0.72 0.83 0.87 0.89 0.9 0.89 0.89 0.72 0.83 0.87 0.88 0.9 0.89 0.89 0.71 0.83 0.87 0.88 0.9 0.89 0.89 0.71 0.83 0.86 0.88 0.9 0.89 0.89 0.7 0.82 0.86 0.88 0.9 0.89 0.89 0.69 0.82 0.86 0.88 0.9 0.89 0.89 0.67 0.81 0.86 0.88 0.9 0.89 0.89 0.63 0.79 0.85 0.87 0.89 0.89 0.89 0.82 0.87 0.88 0.89 0.89 0.89 0.89 0.81 0.87 0.89 0.89 0.9 0.9 0.89 0.76 0.85 0.87 0.89 0.9 0.89 0.89 0.72 0.83 0.86 0.88 0.89 0.89 0.89 0.72 0.83 0.86 0.88 0.89 0.9 0.89 0.71 0.82 0.86 0.88 0.89 0.9 ...(+1314 chars))  G_o=0  omega_o=0  omegaN_o=0  tau_s=.01  maxAbsSpd=5e3  aMode=aMode
  Ideal Fixed Gear Transmission B : autolibsharedtransfixedgear/Ideal Fixed Gear Transmission  VariantControl=0  TransEffModelPopup=Gear only  gearInterp=Nearest  G=[-1, 0, 2, 4, 6, 8]  Trq_bpts=[25, 50, 75, 100, 150, 200, 250]  omega_bpts=[52.4 78.5 105 131 157 183 209 262 314 419 524]  Temp_bpts=[313 358]  N=[N(1), N(2:2:end)]  Jout="[0.28 0.14 0.24 0.18  0.11  0.11]"  bout=[0.003,0.001,0.0025,0.001,0.001,0.001]  eta=[0.9, 0.9, 0.9, 0.95, 0.95,0.95]  eta_tbl=reshape([0.53 0.71 0.77 0.79 0.82 0.82 0.82 0.5 0.7 0.77 0.79 0.82 0.82 0.82 0.54 0.72 0.78 0.81 0.83 0.82 0.82 0.56 0.73 0.79 0.81 0.84 0.82 0.82 0.58 0.74 0.79 0.82 0.84 0.82 0.82 0.57 0.74 0.79 0.82 0.84 0.82 0.82 0.58 0.74 0.79 0.82 0.84 0.82 0.82 0.58 0.74 0.79 0.82 0.84 0.82 0.82 0.57 0.74 0.8 0.82 0.85 0.82 0.82 0.55 0.73 0.78 0.81 0.84 0.82 0.82 0.51 0.71 0.77 0.81 0.84 0.82 0.82 0.53 0.71 0.77 0.79 0.82 0.82 0.82 0.5 0.7 0.77 0.79 0.82 0.82 0.82 0.54 0.72 0.78 0.81 0.83 0.82 0.82 0.56 0.73 0.79 0.81 0.84 0.82 0.82 0.58 0.74 0.79 0.82 0.84 0.82 0.82 0.57 0.74 0.79 0.82 0.84 0.82 0.82 0.58 0.74 0.79 0.82 0.84 0.82 0.82 0.58 0.74 0.79 0.82 0.84 0.82 0.82 0.57 0.74 0.8 0.82 0.85 0.82 0.82 0.55 0.73 0.78 0.81 0.84 0.82 0.82 0.51 0.71 0.77 0.81 0.84 0.82 0.82 0.53 0.71 0.77 0.79 0.82 0.82 0.82 0.5 0.7 0.77 0.79 0.82 0.82 0.82 0.54 0.72 0.78 0.81 0.83 0.82 0.82 0.56 0.73 0.79 0.81 0.84 0.82 0.82 0.58 0.74 0.79 0.82 0.84 0.82 0.82 0.57 0.74 0.79 0.82 0.84 0.82 0.82 0.58 0.74 0.79 0.82 0.84 0.82 0.82 0.58 0.74 0.79 0.82 0.84 0.82 0.82 0.57 0.74 0.8 0.82 0.85 0.82 0.82 0.55 0.73 0.78 0.81 0.84 0.82 0.82 0.51 0.71 0.77 0.81 0.84 0.82 0.82 0.7 0.79 0.82 0.83 0.84 0.84 0.84 0.63 0.76 0.8 0.82 0.83 0.84 0.84 0.58 0.74 0.79 0.81 0.83 0.84 0.84 0.58 0.74 0.79 0.81 0.83 0.84 0.84 0.58 0.74 0.79 0.81 0.84 0.84 0.84 0.57 0.73 0.78 0.81 0.84 0.85 0.84 0.57 0.73 0.79 0.81 0.84 0.85 0.84 0.56 0.73 0.78 0.81 0.83 0.85 0.84 0.55 0.73 0.78 0.81 0.84 0.85 0.84 0.52 0.71 0.77 0.8 0.83 0.85 0.84 0.48 0.69 0.76 0.79 0.83 0.84 0.84 0.64 0.76 0.8 0.81 0.83 0.84 0.84 0.56 0.73 0.78 0.8 0.83 0.84 0.84 0.54 0.71 0.77 0.8 0.82 0.84 0.84 0.53 0.71 0.77 0.8 0.83 0.84 0.84 0.51 0.71 0.77 0.8 0.83 0.84 0.85 0.52 0.7 0.77 0.8 0.83 0.84 0.85 0.51 0.71 0.76 0.79 0.83 0.84 0.85 0.5 0.69 0.76 0.79 0.82 0.84 0.85 0.45 0.68 0.75 0.78 0.82 0.84 0.85 0.43 0.67 0.74 0.78 0.81 0.83 0.84 0.38 0.63 0.71 0.75 0.8 0.82 0.83 0.65 0.79 0.84 0.85 0.88 0.89 0.89 0.56 0.75 0.81 0.83 0.86 0.88 0.89 0.52 0.72 0.79 0.83 0.86 0.88 0.88 0.51 0.72 0.79 0.83 0.86 0.88 0.89 0.49 0.71 0.78 0.82 0.86 0.88 0.89 0.47 0.7 0.78 0.82 0.86 0.87 0.88 0.45 0.69 0.77 0.81 0.85 0.87 0.88 0.4 0.67 0.75 0.8 0.84 0.86 0.88 0.3 0.64 0.73 0.78 0.83 0.86 0.87 0.17 0.55 0.67 0.73 0.8 0.83 0.85 0.089 0.45 0.61 0.69 0.77 0.81 0.83 0.61 0.75 0.82 0.84 0.87 0.87 0.88 0.54 0.73 0.8 0.82 0.86 0.87 0.88 0.51 0.71 0.79 0.82 0.86 0.87 0.88 0.52 0.72 0.79 0.82 0.86 0.87 0.89 0.52 0.72 0.8 0.83 0.86 0.88 0.89 0.53 0.72 0.79 0.82 0.86 0.87 0.89 0.5 0.7 0.78 0.82 0.86 0.88 0.88 0.46 0.69 0.77 0.81 0.85 0.87 0.88 0.4 0.67 0.75 0.8 0.83 0.86 0.88 0.33 0.64 0.73 0.78 0.83 0.85 0.87 0.33 0.64 0.73 0.78 0.83 0.85 0.87 0.78 0.85 0.87 0.88 0.89 0.89 0.89 0.73 0.83 0.86 0.88 0.89 0.89 0.89 0.72 0.83 0.86 0.88 0.89 0.89 0.89 0.72 0.83 0.87 0.89 0.9 0.89 0.89 0.72 0.83 0.87 0.88 0.9 0.89 0.89 0.71 0.83 0.87 0.88 0.9 0.89 0.89 0.71 0.83 0.86 0.88 0.9 0.89 0.89 0.7 0.82 0.86 0.88 0.9 0.89 0.89 0.69 0.82 0.86 0.88 0.9 0.89 0.89 0.67 0.81 0.86 0.88 0.9 0.89 0.89 0.63 0.79 0.85 0.87 0.89 0.89 0.89 0.78 0.85 0.87 0.88 0.89 0.89 0.89 0.73 0.83 0.86 0.88 0.89 0.89 0.89 0.72 0.83 0.86 0.88 0.89 0.89 0.89 0.72 0.83 0.87 0.89 0.9 0.89 0.89 0.72 0.83 0.87 0.88 0.9 0.89 0.89 0.71 0.83 0.87 0.88 0.9 0.89 0.89 0.71 0.83 0.86 0.88 0.9 0.89 0.89 0.7 0.82 0.86 0.88 0.9 0.89 0.89 0.69 0.82 0.86 0.88 0.9 0.89 0.89 0.67 0.81 0.86 0.88 0.9 0.89 0.89 0.63 0.79 0.85 0.87 0.89 0.89 0.89 0.78 0.85 0.87 0.88 0.89 0.89 0.89 0.73 0.83 0.86 0.88 0.89 0.89 0.89 0.72 0.83 0.86 0.88 0.89 0.89 0.89 0.72 0.83 0.87 0.89 0.9 0.89 0.89 0.72 0.83 0.87 0.88 0.9 0.89 0.89 0.71 0.83 0.87 0.88 0.9 0.89 0.89 0.71 0.83 0.86 0.88 0.9 0.89 0.89 0.7 0.82 0.86 0.88 0.9 0.89 0.89 0.69 0.82 0.86 0.88 0.9 0.89 0.89 0.67 0.81 0.86 0.88 0.9 0.89 0.89 0.63 0.79 0.85 0.87 0.89 0.89 0.89 0.82 0.87 0.88 0.89 0.89 0.89 0.89 0.81 0.87 0.89 0.89 0.9 0.9 0.89 0.76 0.85 0.87 0.89 0.9 0.89 0.89 0.72 0.83 0.86 0.88 0.89 0.89 0.89 0.72 0.83 0.86 0.88 0.89 0.9 0.89 0.71 0.82 0.86 0.88 0.89 0.9 ...(+1314 chars))  G_o=0  omega_o=0  omegaN_o=0  tau_s=.01  maxAbsSpd=5e3  aMode=aMode
  Split Torsional Compliance : autolibsharedcoupling/Split Torsional Compliance  port_config=Simulink  cplrMode=Shaft merge  extInfo=off  k1=5e3  b1=b_driveshaft  omega1_c=200  theta1_o=0  domega1_o=0  k2=5e3  b2=b_driveshaft  omega2_c=200  theta2_o=0  domega2_o=0  blkID=0  aMode=1
      settings: LibrarySourceBlock=autolibcoupling/Split Torsional Compliance
  Torsional Compliance : autolibsharedcoupling/Torsional Compliance  port_config=Two-way connection  extInfo=off  k=k_driveshaft  b=b_driveshaft  theta_o=0  domega_o=0  omega_c=wc_shaft  blkID=0  aMode=1
  Torsional Compliance1 : autolibsharedcoupling/Torsional Compliance  port_config=Two-way connection  extInfo=off  k=k_driveshaft  b=b_driveshaft  theta_o=0  domega_o=0  omega_c=wc_shaft  blkID=0  aMode=1
  Two-Way Connection2 : TwoWayConnection
  Two-Way Connection3 : TwoWayConnection
  Two-Way Connection4 : TwoWayConnection
  A Clutch : PMIOPort  Side=Left
  B Clutch : PMIOPort  Port=2  Side=Left
  T : PMIOPort  Port=3  Side=Right
  A Gears Info : Outport  VectorParamsAs1DForOutWhenUnconnected=off
  B Gears Info : Outport  Port=2  VectorParamsAs1DForOutWhenUnconnected=off
  T_Out : Outport  Port=3  VectorParamsAs1DForOutWhenUnconnected=off
  w_Out : Outport  Port=4  VectorParamsAs1DForOutWhenUnconnected=off
  wires:
  Ideal Fixed Gear Transmission B/1 -> B Gears Info/1
  Ideal Fixed Gear Transmission A/1 -> A Gears Info/1
  Ideal Fixed Gear Transmission B/2 -> Two-Way Connection3/1
  Gear Coord/2(B) -> Ideal Fixed Gear Transmission B/1
  Two-Way Connection2/1 -> Ideal Fixed Gear Transmission A/2
  Gear Cmd/1 -> Gear Coord/1(In1)
  Gear Coord/1(A) -> Ideal Fixed Gear Transmission A/1
  Two-Way Connection3/1 -> Ideal Fixed Gear Transmission B/2
  Ideal Fixed Gear Transmission A/2 -> Two-Way Connection2/1
  Ideal Fixed Gear Transmission B/3 -> Split Torsional Compliance/3
  Split Torsional Compliance/1 -> Two-Way Connection4/1, T_Out/1
  Two-Way Connection4/1 -> Split Torsional Compliance/1, w_Out/1
  Ideal Fixed Gear Transmission A/3 -> Split Torsional Compliance/2
  Split Torsional Compliance/3 -> Ideal Fixed Gear Transmission B/3
  Split Torsional Compliance/2 -> Ideal Fixed Gear Transmission A/3
  connections:
  Torsional Compliance1/LConn1 -- B Clutch/RConn1
  Torsional Compliance/RConn1 -- Two-Way Connection2/RConn1
  Torsional Compliance1/RConn1 -- Two-Way Connection3/RConn1
  Torsional Compliance/LConn1 -- A Clutch/RConn1
  Two-Way Connection4/RConn1 -- T/RConn1

== system DrivetrainConVeh/DCT/DCT System/Hydraulics ==
  Gear Cmd : Inport
  A Cmd : Inport  Port=2
  B Cmd : Inport  Port=3
  A Hydraulics Tau : Subsystem
  B Hydraulics Tau : Subsystem
  A Press : Outport  VectorParamsAs1DForOutWhenUnconnected=off
  B Press : Outport  Port=2  VectorParamsAs1DForOutWhenUnconnected=off
  wires:
  B Hydraulics Tau/1(Out1) -> B Press/1
  Gear Cmd/1 -> B Hydraulics Tau/1(In1), A Hydraulics Tau/1(In1)
  A Hydraulics Tau/1(Out1) -> A Press/1
  A Cmd/1 -> A Hydraulics Tau/2(In2)
  B Cmd/1 -> B Hydraulics Tau/2(In2)

== system DrivetrainConVeh/Differential and Compliance/All Wheel Drive/Front Axle Compliance 2 ==
  Info : Inport
  Bus Selector : BusSelector  OutputSignals=PwrInfo.PwrTrnsfrd,PwrInfo.PwrNotTrnsfrd,PwrInfo.PwrStored
  Bus Selector1 : BusSelector  OutputSignals=Trq.R,Trq.C
  Power Accounting Bus Creator : autolibpowerinfoutils/Power Accounting Bus Creator  AssctBlkSelPopup=Parent  RefBlkName='libraryname/blkname'  PwrTrnsfrdCheckBox=on  PwrNotTrnsfrdCheckBox=on  PwrStoredCheckBox=on  aMode=aMode
  Terminator : Terminator
  Terminator1 : Terminator
  Terminator2 : Terminator
  Two-Way Connection1 : TwoWayConnection
  Two-Way Connection4 : TwoWayConnection
  R : PMIOPort  Side=Left
  C : PMIOPort  Port=2  Side=Right
  wires:
  Two-Way Connection4/1 -> Terminator/1
  Info/1 -> Bus Selector1/1, Bus Selector/1
  Two-Way Connection1/1 -> Terminator1/1
  Bus Selector1/1 -> Two-Way Connection4/1  "<R>"
  Bus Selector1/2 -> Two-Way Connection1/1  "<C>"
  Power Accounting Bus Creator/1 -> Terminator2/1
  Bus Selector/1 -> Power Accounting Bus Creator/1  "<PwrTrnsfrd>"
  Bus Selector/2 -> Power Accounting Bus Creator/2  "<PwrNotTrnsfrd>"
  Bus Selector/3 -> Power Accounting Bus Creator/3  "<PwrStored>"
  connections:
  R/RConn1 -- Two-Way Connection4/RConn1
  Two-Way Connection1/RConn1 -- C/RConn1

== system DrivetrainConVeh/Differential and Compliance/All Wheel Drive/Rear Axle Compliance 2 ==
  Info : Inport
  Bus Selector : BusSelector  OutputSignals=PwrInfo.PwrTrnsfrd,PwrInfo.PwrNotTrnsfrd,PwrInfo.PwrStored
  Bus Selector1 : BusSelector  OutputSignals=Trq.R,Trq.C
  Power Accounting Bus Creator : autolibpowerinfoutils/Power Accounting Bus Creator  AssctBlkSelPopup=Parent  RefBlkName='libraryname/blkname'  PwrTrnsfrdCheckBox=on  PwrNotTrnsfrdCheckBox=on  PwrStoredCheckBox=on  aMode=aMode
  Terminator : Terminator
  Terminator1 : Terminator
  Terminator2 : Terminator
  Two-Way Connection1 : TwoWayConnection
  Two-Way Connection4 : TwoWayConnection
  R : PMIOPort  Side=Left
  C : PMIOPort  Port=2  Side=Right
  wires:
  Two-Way Connection4/1 -> Terminator/1
  Info/1 -> Bus Selector1/1, Bus Selector/1
  Two-Way Connection1/1 -> Terminator1/1
  Bus Selector1/1 -> Two-Way Connection4/1  "<R>"
  Bus Selector1/2 -> Two-Way Connection1/1  "<C>"
  Power Accounting Bus Creator/1 -> Terminator2/1
  Bus Selector/1 -> Power Accounting Bus Creator/1  "<PwrTrnsfrd>"
  Bus Selector/2 -> Power Accounting Bus Creator/2  "<PwrNotTrnsfrd>"
  Bus Selector/3 -> Power Accounting Bus Creator/3  "<PwrStored>"
  connections:
  R/RConn1 -- Two-Way Connection4/RConn1
  Two-Way Connection1/RConn1 -- C/RConn1
